simulink model "Prueba"  (Simulink 7.7)
settings: Solver=ode45  StartTime=0.0  StopTime=10.0  RelTol=1e-3
settings Model: Creator=alumno  LastModifiedBy=Leonardo

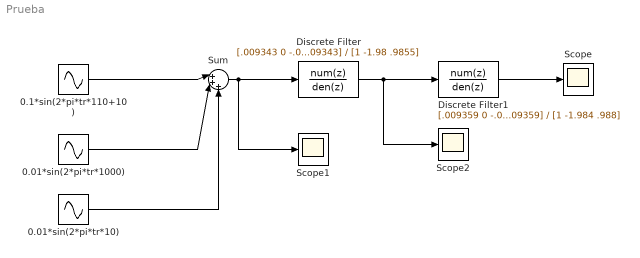
== system Prueba ==
  0.01*sin(2*pi*tr*10) : Sin  Amplitude=.01  Frequency=2*pi*10  SampleTime=0
  0.01*sin(2*pi*tr*1000) : Sin  Amplitude=.01  Frequency=2*pi*1000  SampleTime=0
  0.1*sin(2*pi*tr*110+10) : Sin  Amplitude=.1  Frequency=2*pi*110  Phase=10  SampleTime=0
  Discrete Filter : DiscreteFilter  Numerator=[.009343 0 -.009343]  Denominator=[1 -1.98 .9855]  SampleTime=1/10000
  Discrete Filter1 : DiscreteFilter  Numerator=[.009359 0 -.009359]  Denominator=[1 -1.984 .988]  SampleTime=1/10000
  Scope : Scope
  Scope1 : Scope
  Scope2 : Scope
      settings: SaveName=ScopeData2
  Sum : Sum  Inputs=|+++
  wires:
  0.1*sin(2*pi*tr*110+10)/1 -> Sum/1
  0.01*sin(2*pi*tr*1000)/1 -> Sum/2
  0.01*sin(2*pi*tr*10)/1 -> Sum/3
  Discrete Filter/1 -> Discrete Filter1/1, Scope2/1
  Discrete Filter1/1 -> Scope/1
  Sum/1 -> Scope1/1, Discrete Filter/1
